simulink model "sim1_nonmininumS"  (R2018b)
settings: Solver=VariableStepAuto  StartTime=0.0  StopTime=Tsim  RelTol=1e-3
values from neighbouring files (symbols this model uses):
  Apert = -0.06    [ex3_geng.m]
  Aruido = 0.05    [ex3_geng.m]
  kr = inv(C*inv(eye(2)-A+B*K)*B)    [ex1_liu.m]    (also in ex2_fu.m = inv([1 0]*inv(eye(2)-A+B*K)*B); ex2_liu.m; ex3_geng.m = inv([1 0]*inv(eye(2)-A+B*K)*B); ex3_liu_geso.m = inv([1 0]*inv(eye(2)-A+B*K)*B))
  Pruido = 0.000004    (= 4e-06)    [ex3_geng.m]
  ref = 0.2    [ex3_geng.m]
  Tpert = 20    [ex3_geng.m]
  Truido = 35    [ex3_geng.m]
  Ts = 0.1    [ex1_liu.m]    (also in ex2_fu.m = 0.05; ex2_liu.m; ex3_geng.m = 0.01; gerar_figuras.m)
libraries: cstblocks x4, simulink x1
settings Model: Creator=Bismark  LastModifiedBy=rene
settings DebuggingCC: LibraryContextMissingDiagnostic=none
settings SFSimCC: SimUseLocalCustomCode=off
settings RTWCC: RTWUseLocalCustomCode=off
settings CodeAppCC: StateflowObjectComments=on

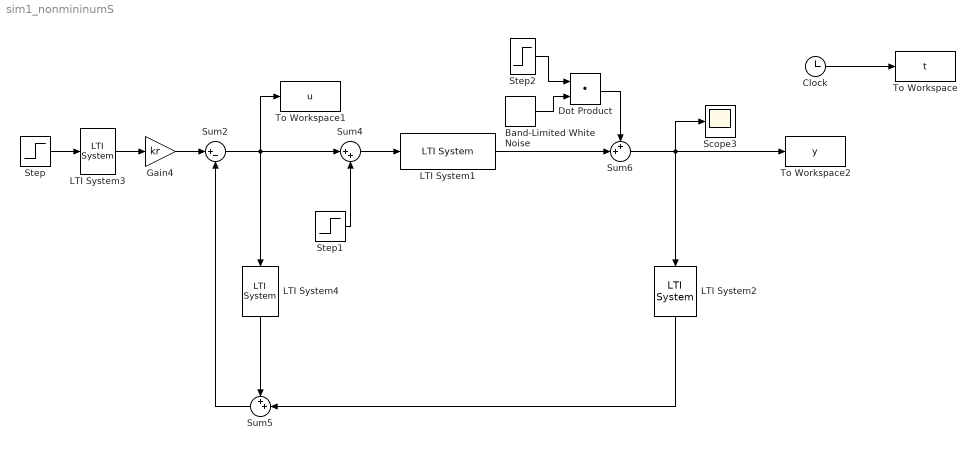
== system sim1_nonmininumS ==
  Band-Limited White Noise : simulink/Sources/Band-Limited White Noise  Cov=[Pruido]  Ts=Ts  seed=[23341]
  Clock : Clock
  Dot Product : DotProduct  InputSameDT=on  OutDataTypeStr=Inherit: Inherit via internal rule
  Gain4 : Gain  Gain=kr
  LTI System1 : cstblocks/LTI System  sys=Pr  IC=[]
  LTI System2 : cstblocks/LTI System  sys=V  IC=[]
  LTI System3 : cstblocks/LTI System  sys=Fr  IC=[]
  LTI System4 : cstblocks/LTI System  sys=S  IC=[]
  Scope3 : Scope
  Step : Step  Time=0  After=ref  SampleTime=0
  Step1 : Step  Time=Tpert  After=Apert  SampleTime=Ts
  Step2 : Step  Time=Truido  After=Aruido  SampleTime=0
  Sum2 : Sum  Inputs=|+-
  Sum4 : Sum  Inputs=|++
  Sum5 : Sum  Inputs=++|
  Sum6 : Sum  Inputs=++|
  To Workspace : ToWorkspace  VariableName=t  SampleTime=Ts
  To Workspace1 : ToWorkspace  VariableName=u  SampleTime=Ts
  To Workspace2 : ToWorkspace  VariableName=y  SampleTime=Ts
  wires:
  Step/1 -> LTI System3/1
  Sum2/1 -> To Workspace1/1, Sum4/1, LTI System4/1
  Gain4/1 -> Sum2/1
  Clock/1 -> To Workspace/1
  Sum4/1 -> LTI System1/1
  Step1/1 -> Sum4/2
  Sum5/1 -> Sum2/2
  Sum6/1 -> Scope3/1, To Workspace2/1, LTI System2/1
  LTI System2/1 -> Sum5/2
  LTI System3/1 -> Gain4/1
  Step2/1 -> Dot Product/1
  Band-Limited White Noise/1 -> Dot Product/2
  LTI System4/1 -> Sum5/1
  Dot Product/1 -> Sum6/1
  LTI System1/1 -> Sum6/2
